simulink model "Final_Model"  (R2022b)
settings: Solver=FixedStepAuto  StartTime=0.0  StopTime=5  FixedStep=0.001  RelTol=1e-3
model workspace: external: MATLAB File F:\Iman\Robotics\Project1\solid_simmmmm\Final_Model_DataFile.m (data not in the file)
undefined symbols (not defined in the file or in its folder): Revolute, Revolute3, Revolute4, smiData, X, Y, Z
libraries: sm_lib x139, nesl_utility x53
(part 4 of 4)

== system Final_Model/IK/Link1_2_RIGID ==
  ReferenceFrame : sm_lib/Frames and Transforms/Reference Frame
  Solid : sm_lib/Body Elements/File Solid  ExtGeomFileName=Link1_Default_sldprt.STEP  UnitType=FromFile  ExtGeomFileUnits=m  StepReaderType=HEX  ExportConvexHullGeometry=off  InertiaType=Custom  Mass=smiData.Solid(3).mass  MassUnits=kg  CenterOfMass=smiData.Solid(3).CoM  CenterOfMassUnits=m  MomentsOfInertia=smiData.Solid(3).MoI  MomentsOfInertiaUnits=kg*m^2  ProductsOfInertia=smiData.Solid(3).PoI  ProductsOfInertiaUnits=kg*m^2  BasedOnType=DensityFromFile  Density=1000  DensityUnits=kg/m^3  DoExposeReferenceFrame=on  SerializedFrames=<Frames/>  GraphicType=FromGeometry  MarkerShape=Sphere  MarkerSize=10  GraphicVisPropType=SimpleVisualProperties  GraphicDiffuseColor=smiData.Solid(3).color  GraphicSpecularColor=[0.5 0.5 0.5 1.0]  GraphicAmbientColor=[0.15 0.15 0.15 1.0]  GraphicEmissiveColor=[0.0 0.0 0.0 1.0]  GraphicShininess=75  GraphicOpacity=smiData.Solid(3).opacity
  Transform : sm_lib/Frames and Transforms/Rigid Transform  TranslationMethod=Cartesian  TranslationStandardOffset=0  TranslationLengthUnit=cm  TranslationStandardAxis=+Z  TranslationCartesianOffset=smiData.RigidTransform(6).translation  TranslationROffset=0  TranslationROffsetUnits=m  TranslationZOffset=0  TranslationZOffsetUnits=m  TranslationThetaOffset=0  TranslationThetaOffsetUnits=deg  RotationMethod=ArbitraryAxis  RotationAngleUnits=rad  RotationStandardAxis=+Z  RotationAngle=smiData.RigidTransform(6).angle  RotationArbitraryAxis=smiData.RigidTransform(6).axis  FollAlignAxisA=+X  BaseAlignAxisA=+Y  FollAlignAxisB=+Y  BaseAlignAxisB=+Z  RotationSequenceAxes=FollowerAxes  RotationSequence=XYX  RotationSequenceAngles=[0 0 0]  RotationSequenceAnglesUnits=deg  RotationMatrix=[1 0 0; 0 1 0; 0 0 1]  Quaternion=[1 0 0 0]
  Transform1 : sm_lib/Frames and Transforms/Rigid Transform  TranslationMethod=Cartesian  TranslationStandardOffset=0  TranslationLengthUnit=cm  TranslationStandardAxis=+Z  TranslationCartesianOffset=smiData.RigidTransform(7).translation  TranslationROffset=0  TranslationROffsetUnits=m  TranslationZOffset=0  TranslationZOffsetUnits=m  TranslationThetaOffset=0  TranslationThetaOffsetUnits=deg  RotationMethod=ArbitraryAxis  RotationAngleUnits=rad  RotationStandardAxis=+Z  RotationAngle=smiData.RigidTransform(7).angle  RotationArbitraryAxis=smiData.RigidTransform(7).axis  FollAlignAxisA=+X  BaseAlignAxisA=+Y  FollAlignAxisB=+Y  BaseAlignAxisB=+Z  RotationSequenceAxes=FollowerAxes  RotationSequence=XYX  RotationSequenceAngles=[0 0 0]  RotationSequenceAnglesUnits=deg  RotationMatrix=[1 0 0; 0 1 0; 0 0 1]  Quaternion=[1 0 0 0]
  F : PMIOPort  Side=Left
  F1 : PMIOPort  Port=2  Side=Right
  connections:
  Solid/RConn1 -- ReferenceFrame/RConn1 -- Transform/LConn1 -- Transform1/LConn1
  Transform/RConn1 -- F/RConn1
  Transform1/RConn1 -- F1/RConn1

== system Final_Model/IK/Link2_1_RIGID ==
  ReferenceFrame : sm_lib/Frames and Transforms/Reference Frame
  Solid : sm_lib/Body Elements/File Solid  ExtGeomFileName=Link2_Default_sldprt.STEP  UnitType=FromFile  ExtGeomFileUnits=m  StepReaderType=HEX  ExportConvexHullGeometry=off  InertiaType=Custom  Mass=smiData.Solid(4).mass  MassUnits=kg  CenterOfMass=smiData.Solid(4).CoM  CenterOfMassUnits=m  MomentsOfInertia=smiData.Solid(4).MoI  MomentsOfInertiaUnits=kg*m^2  ProductsOfInertia=smiData.Solid(4).PoI  ProductsOfInertiaUnits=kg*m^2  BasedOnType=DensityFromFile  Density=1000  DensityUnits=kg/m^3  DoExposeReferenceFrame=on  SerializedFrames=<Frames/>  GraphicType=FromGeometry  MarkerShape=Sphere  MarkerSize=10  GraphicVisPropType=SimpleVisualProperties  GraphicDiffuseColor=smiData.Solid(4).color  GraphicSpecularColor=[0.5 0.5 0.5 1.0]  GraphicAmbientColor=[0.15 0.15 0.15 1.0]  GraphicEmissiveColor=[0.0 0.0 0.0 1.0]  GraphicShininess=75  GraphicOpacity=smiData.Solid(4).opacity
  Transform : sm_lib/Frames and Transforms/Rigid Transform  TranslationMethod=Cartesian  TranslationStandardOffset=0  TranslationLengthUnit=cm  TranslationStandardAxis=+Z  TranslationCartesianOffset=smiData.RigidTransform(5).translation  TranslationROffset=0  TranslationROffsetUnits=m  TranslationZOffset=0  TranslationZOffsetUnits=m  TranslationThetaOffset=0  TranslationThetaOffsetUnits=deg  RotationMethod=ArbitraryAxis  RotationAngleUnits=rad  RotationStandardAxis=+Z  RotationAngle=smiData.RigidTransform(5).angle  RotationArbitraryAxis=smiData.RigidTransform(5).axis  FollAlignAxisA=+X  BaseAlignAxisA=+Y  FollAlignAxisB=+Y  BaseAlignAxisB=+Z  RotationSequenceAxes=FollowerAxes  RotationSequence=XYX  RotationSequenceAngles=[0 0 0]  RotationSequenceAnglesUnits=deg  RotationMatrix=[1 0 0; 0 1 0; 0 0 1]  Quaternion=[1 0 0 0]
  Transform1 : sm_lib/Frames and Transforms/Rigid Transform  TranslationMethod=Cartesian  TranslationStandardOffset=0  TranslationLengthUnit=cm  TranslationStandardAxis=+Z  TranslationCartesianOffset=smiData.RigidTransform(9).translation  TranslationROffset=0  TranslationROffsetUnits=m  TranslationZOffset=0  TranslationZOffsetUnits=m  TranslationThetaOffset=0  TranslationThetaOffsetUnits=deg  RotationMethod=ArbitraryAxis  RotationAngleUnits=rad  RotationStandardAxis=+Z  RotationAngle=smiData.RigidTransform(9).angle  RotationArbitraryAxis=smiData.RigidTransform(9).axis  FollAlignAxisA=+X  BaseAlignAxisA=+Y  FollAlignAxisB=+Y  BaseAlignAxisB=+Z  RotationSequenceAxes=FollowerAxes  RotationSequence=XYX  RotationSequenceAngles=[0 0 0]  RotationSequenceAnglesUnits=deg  RotationMatrix=[1 0 0; 0 1 0; 0 0 1]  Quaternion=[1 0 0 0]
  F : PMIOPort  Side=Right
  F1 : PMIOPort  Port=2  Side=Right
  connections:
  Solid/RConn1 -- ReferenceFrame/RConn1 -- Transform/LConn1 -- Transform1/LConn1
  Transform/RConn1 -- F/RConn1
  Transform1/RConn1 -- F1/RConn1

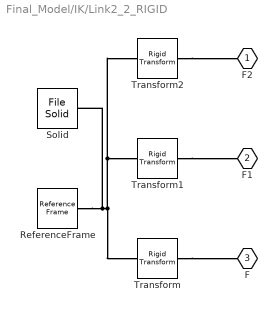
== system Final_Model/IK/Link2_2_RIGID ==
  ReferenceFrame : sm_lib/Frames and Transforms/Reference Frame
  Solid : sm_lib/Body Elements/File Solid  ExtGeomFileName=Link2_Default_sldprt.STEP  UnitType=FromFile  ExtGeomFileUnits=m  StepReaderType=HEX  ExportConvexHullGeometry=off  InertiaType=Custom  Mass=smiData.Solid(4).mass  MassUnits=kg  CenterOfMass=smiData.Solid(4).CoM  CenterOfMassUnits=m  MomentsOfInertia=smiData.Solid(4).MoI  MomentsOfInertiaUnits=kg*m^2  ProductsOfInertia=smiData.Solid(4).PoI  ProductsOfInertiaUnits=kg*m^2  BasedOnType=DensityFromFile  Density=1000  DensityUnits=kg/m^3  DoExposeReferenceFrame=on  SerializedFrames=<Frames/>  GraphicType=FromGeometry  MarkerShape=Sphere  MarkerSize=10  GraphicVisPropType=SimpleVisualProperties  GraphicDiffuseColor=smiData.Solid(4).color  GraphicSpecularColor=[0.5 0.5 0.5 1.0]  GraphicAmbientColor=[0.15 0.15 0.15 1.0]  GraphicEmissiveColor=[0.0 0.0 0.0 1.0]  GraphicShininess=75  GraphicOpacity=smiData.Solid(4).opacity
  Transform : sm_lib/Frames and Transforms/Rigid Transform  TranslationMethod=Cartesian  TranslationStandardOffset=0  TranslationLengthUnit=cm  TranslationStandardAxis=+Z  TranslationCartesianOffset=smiData.RigidTransform(2).translation  TranslationROffset=0  TranslationROffsetUnits=m  TranslationZOffset=0  TranslationZOffsetUnits=m  TranslationThetaOffset=0  TranslationThetaOffsetUnits=deg  RotationMethod=ArbitraryAxis  RotationAngleUnits=rad  RotationStandardAxis=+Z  RotationAngle=smiData.RigidTransform(2).angle  RotationArbitraryAxis=smiData.RigidTransform(2).axis  FollAlignAxisA=+X  BaseAlignAxisA=+Y  FollAlignAxisB=+Y  BaseAlignAxisB=+Z  RotationSequenceAxes=FollowerAxes  RotationSequence=XYX  RotationSequenceAngles=[0 0 0]  RotationSequenceAnglesUnits=deg  RotationMatrix=[1 0 0; 0 1 0; 0 0 1]  Quaternion=[1 0 0 0]
  Transform1 : sm_lib/Frames and Transforms/Rigid Transform  TranslationMethod=Cartesian  TranslationStandardOffset=0  TranslationLengthUnit=cm  TranslationStandardAxis=+Z  TranslationCartesianOffset=smiData.RigidTransform(8).translation  TranslationROffset=0  TranslationROffsetUnits=m  TranslationZOffset=0  TranslationZOffsetUnits=m  TranslationThetaOffset=0  TranslationThetaOffsetUnits=deg  RotationMethod=ArbitraryAxis  RotationAngleUnits=rad  RotationStandardAxis=+Z  RotationAngle=smiData.RigidTransform(8).angle  RotationArbitraryAxis=smiData.RigidTransform(8).axis  FollAlignAxisA=+X  BaseAlignAxisA=+Y  FollAlignAxisB=+Y  BaseAlignAxisB=+Z  RotationSequenceAxes=FollowerAxes  RotationSequence=XYX  RotationSequenceAngles=[0 0 0]  RotationSequenceAnglesUnits=deg  RotationMatrix=[1 0 0; 0 1 0; 0 0 1]  Quaternion=[1 0 0 0]
  Transform2 : sm_lib/Frames and Transforms/Rigid Transform  TranslationMethod=Cartesian  TranslationStandardOffset=0  TranslationLengthUnit=cm  TranslationStandardAxis=+Z  TranslationCartesianOffset=smiData.RigidTransform(11).translation  TranslationROffset=0  TranslationROffsetUnits=m  TranslationZOffset=0  TranslationZOffsetUnits=m  TranslationThetaOffset=0  TranslationThetaOffsetUnits=deg  RotationMethod=ArbitraryAxis  RotationAngleUnits=rad  RotationStandardAxis=+Z  RotationAngle=smiData.RigidTransform(11).angle  RotationArbitraryAxis=smiData.RigidTransform(11).axis  FollAlignAxisA=+X  BaseAlignAxisA=+Y  FollAlignAxisB=+Y  BaseAlignAxisB=+Z  RotationSequenceAxes=FollowerAxes  RotationSequence=XYX  RotationSequenceAngles=[0 0 0]  RotationSequenceAnglesUnits=deg  RotationMatrix=[1 0 0; 0 1 0; 0 0 1]  Quaternion=[1 0 0 0]
  F2 : PMIOPort  Side=Left
  F1 : PMIOPort  Port=2  Side=Left
  F : PMIOPort  Port=3  Side=Left
  connections:
  Solid/RConn1 -- ReferenceFrame/RConn1 -- Transform1/LConn1 -- Transform2/LConn1 -- Transform/LConn1
  Transform/RConn1 -- F/RConn1
  Transform1/RConn1 -- F1/RConn1
  Transform2/RConn1 -- F2/RConn1

== matlab function Final_Model/Rev3 Trajectory/Rev3 trajectories2 ==
  data: t input; theta0 input; pos3 output; thetaf input; thetad0 input; thetadf input; thetadd0 input; thetaddf input; tstart input; pos5 output; tfinal input
function [pos3, pos5] = fcn(t, theta0, thetaf, thetad0, thetadf, thetadd0, thetaddf, tstart, tfinal)
    % Input parameters:
    % t         - current time from Simulink clock
    % theta0    - initial position
    % thetaf    - final position
    % thetad0   - initial velocity
    % thetadf   - final velocity
    % thetadd0  - initial acceleration (for 5th order only)
    % thetaddf  - final acceleration (for 5th order only)
    % tstart    - start time
    % tfinal    - final time
    
    % Outputs:
    % pos3      - position from 3rd order trajectory
    % pos5      - position from 5th order trajectory
    
    % Calculate time duration
    T = tfinal - tstart;
    
    % 3rd order trajectory coefficients
    a0_3 = theta0;
    a1_3 = thetad0;
    a2_3 = (-3 * (theta0 - thetaf) - (2 * thetad0 + thetadf) * T) / T^2;
    a3_3 = (2 * (theta0 - thetaf) + (thetad0 + thetadf) * T) / T^3;
    
    % 5th order trajectory coefficients
    a0_5 = theta0;
    a1_5 = thetad0;
    a2_5 = 0.5 * thetadd0;
    a3_5 = (1/(2*T^3)) * (20 * (thetaf - theta0) - (8 * thetadf + 12*thetad0) * T - (3 * thetaddf - thetadd0) * T^2);
    a4_5 = (1/(2*T^4)) * (30 * (theta0 - thetaf) + (14 * thetadf + 16*thetad0) * T + (3 * thetaddf - 2*thetadd0) * T^2);
    a5_5 = (1/(2*T^5)) * (12 * (thetaf - theta0) - 6*(thetadf + thetad0) * T - (thetaddf - thetadd0) * T^2);
    
    % Calculate relative time
    t_rel = t - tstart;
    
    % Ensure trajectory stays at final position after tfinal
    if t < tstart
        pos3 = theta0;
        pos5 = theta0;
    elseif t > tfinal
        pos3 = thetaf;
        pos5 = thetaf;
    else
        % Calculate positions using polynomial equations
        pos3 = a0_3 + a1_3*t_rel + a2_3*t_rel^2 + a3_3*t_rel^3;
        pos5 = a0_5 + a1_5*t_rel + a2_5*t_rel^2 + a3_5*t_rel^3 + a4_5*t_rel^4 + a5_5*t_rel^5;
    end
end

== matlab function Final_Model/Multiply ==
  data: u input; y1 output; v input; y2 output; y3 output
function [y1, y2, y3] = power(u,v)

y1 = u(1) * v(1);
y2 = u(2) * v(2);
y3 = u(3) * v(3);

== matlab function Final_Model/MATLAB Function1 ==
  data: t input; y output
function y = fcn(t)

y = 30 * sin(t) + 45; %theta2

== matlab function Final_Model/MATLAB Function ==
  data: t input; y output
function y = fcn(t)

y = 30 * sin(t); %theta1

== matlab function Final_Model/MATLAB Function2 ==
  data: t input; y output
function y = fcn(t)

y = 22.5 * sin(t) + 135 ; %theta3

== matlab function Final_Model/MATLAB Function3 ==
  data: t input; y output
function y = fcn(t)

y = 30 * sin(t); %theta1

== matlab function Final_Model/MATLAB Function4 ==
  data: t input; y output
function y = fcn(t)

y = 30 * sin(t) + 45; %theta2

== matlab function Final_Model/MATLAB Function5 ==
  data: t input; y output
function y = fcn(t)

y = 22.5 * sin(t) + 135 ; %theta3

== matlab function Final_Model/MATLAB Function6 ==
  data: x0 input; traj3 output; xf input; v0 input; vf input; a0 input; af input; T input; traj5 output; coeff3 output; coeff5 output; t input
function [traj3, traj5, coeff3, coeff5] = generateTrajectory(x0, xf, v0, vf, a0, af, T,t)
% GENERATETRAJECTORY Generates 3rd and 5th order trajectories.
% 
% Inputs:
%   x0  - Initial position
%   xf  - Final position
%   v0  - Initial velocity
%   vf  - Final velocity
%   a0  - Initial acceleration
%   af  - Final acceleration
%   T   - Total time for the trajectory
%   N   - Number of points for time discretization
% 
% Outputs:
%   traj3  - 3rd order trajectory positions
%   traj5  - 5th order trajectory positions
%   coeff3 - Coefficients of the 3rd order polynomial
%   coeff5 - Coefficients of the 5th order polynomial
%   t      - Time vector
%N = 1;
    % Time vector
    %t = linspace(0, T, N);

    % 3rd-Order Polynomial Coefficients
    A3 = [1, 0, 0, 0; 
          1, T, T^2, T^3; 
          0, 1, 0, 0; 
          0, 1, 2*T, 3*T^2];
    B3 = [x0; xf; v0; vf];
    coeff3 = A3 \ B3;

    % Evaluate 3rd order trajectory
    traj3 = coeff3(1) + coeff3(2)*t + coeff3(3)*t.^2 + coeff3(4)*t.^3;

    % 5th-Order Polynomial Coefficients
    A5 = [1, 0, 0, 0, 0, 0; 
          1, T, T^2, T^3, T^4, T^5; 
          0, 1, 0, 0, 0, 0; 
          0, 1, 2*T, 3*T^2, 4*T^3, 5*T^4; 
          0, 0, 2, 0, 0, 0; 
          0, 0, 2, 6*T, 12*T^2, 20*T^3];
    B5 = [x0; xf; v0; vf; a0; af];
    coeff5 = A5 \ B5;

    % Evaluate 5th order trajectory
    traj5 = coeff5(1) + coeff5(2)*t + coeff5(3)*t.^2 + coeff5(4)*t.^3 + ...
            coeff5(5)*t.^4 + coeff5(6)*t.^5;

%     % Plot the results
%     figure;
%     subplot(2, 1, 1);
%     plot(t, traj3, 'r', 'LineWidth', 2);
%     title('3rd Order Trajectory');
%     xlabel('Time (s)');
%     ylabel('Position (m)');
%     grid on;
% 
%     subplot(2, 1, 2);
%     plot(t, traj5, 'b', 'LineWidth', 2);
%     title('5th Order Trajectory');
%     xlabel('Time (s)');
%     ylabel('Position (m)');
%     grid on;
% 
%     % Display coefficients
%     disp('3rd Order Coefficients:');
%     disp(coeff3);
%     disp('5th Order Coefficients:');
%     disp(coeff5);
end

== matlab function Final_Model/Rev4 Trajectory/Rev4 trajectories ==
  data: t input; theta0 input; pos3 output; thetaf input; thetad0 input; thetadf input; thetadd0 input; thetaddf input; tstart input; pos5 output; tfinal input
function [pos3, pos5] = fcn(t, theta0, thetaf, thetad0, thetadf, thetadd0, thetaddf, tstart, tfinal)
    % Input parameters:
    % t         - current time from Simulink clock
    % theta0    - initial position
    % thetaf    - final position
    % thetad0   - initial velocity
    % thetadf   - final velocity
    % thetadd0  - initial acceleration (for 5th order only)
    % thetaddf  - final acceleration (for 5th order only)
    % tstart    - start time
    % tfinal    - final time
    
    % Outputs:
    % pos3      - position from 3rd order trajectory
    % pos5      - position from 5th order trajectory
    
    % Calculate time duration
    T = tfinal - tstart;
    
    % 3rd order trajectory coefficients
    a0_3 = theta0;
    a1_3 = thetad0;
    a2_3 = (-3 * (theta0 - thetaf) - (2 * thetad0 + thetadf) * T) / T^2;
    a3_3 = (2 * (theta0 - thetaf) + (thetad0 + thetadf) * T) / T^3;
    
    % 5th order trajectory coefficients
    a0_5 = theta0;
    a1_5 = thetad0;
    a2_5 = 0.5 * thetadd0;
    a3_5 = (1/(2*T^3)) * (20 * (thetaf - theta0) - (8 * thetadf + 12*thetad0) * T - (3 * thetaddf - thetadd0) * T^2);
    a4_5 = (1/(2*T^4)) * (30 * (theta0 - thetaf) + (14 * thetadf + 16*thetad0) * T + (3 * thetaddf - 2*thetadd0) * T^2);
    a5_5 = (1/(2*T^5)) * (12 * (thetaf - theta0) - 6*(thetadf + thetad0) * T - (thetaddf - thetadd0) * T^2);
    
    % Calculate relative time
    t_rel = t - tstart;
    
    % Ensure trajectory stays at final position after tfinal
    if t < tstart
        pos3 = theta0;
        pos5 = theta0;
    elseif t > tfinal
        pos3 = thetaf;
        pos5 = thetaf;
    else
        % Calculate positions using polynomial equations
        pos3 = a0_3 + a1_3*t_rel + a2_3*t_rel^2 + a3_3*t_rel^3;
        pos5 = a0_5 + a1_5*t_rel + a2_5*t_rel^2 + a3_5*t_rel^3 + a4_5*t_rel^4 + a5_5*t_rel^5;
    end
end

== matlab function Final_Model/Rev Trajectory/Rev trajectories ==
  data: t input; theta0 input; pos3 output; thetaf input; thetad0 input; thetadf input; thetadd0 input; thetaddf input; tstart input; pos5 output; tfinal input
function [pos3, pos5] = fcn(t, theta0, thetaf, thetad0, thetadf, thetadd0, thetaddf, tstart, tfinal)
    % Input parameters:
    % t         - current time from Simulink clock
    % theta0    - initial position
    % thetaf    - final position
    % thetad0   - initial velocity
    % thetadf   - final velocity
    % thetadd0  - initial acceleration (for 5th order only)
    % thetaddf  - final acceleration (for 5th order only)
    % tstart    - start time
    % tfinal    - final time
    
    % Outputs:
    % pos3      - position from 3rd order trajectory
    % pos5      - position from 5th order trajectory
    
    % Calculate time duration
    T = tfinal - tstart;
    
    % 3rd order trajectory coefficients
    a0_3 = theta0;
    a1_3 = thetad0;
    a2_3 = (-3 * (theta0 - thetaf) - (2 * thetad0 + thetadf) * T) / T^2;
    a3_3 = (2 * (theta0 - thetaf) + (thetad0 + thetadf) * T) / T^3;
    
    % 5th order trajectory coefficients
    a0_5 = theta0;
    a1_5 = thetad0;
    a2_5 = 0.5 * thetadd0;
    a3_5 = (1/(2*T^3)) * (20 * (thetaf - theta0) - (8 * thetadf + 12*thetad0) * T - (3 * thetaddf - thetadd0) * T^2);
    a4_5 = (1/(2*T^4)) * (30 * (theta0 - thetaf) + (14 * thetadf + 16*thetad0) * T + (3 * thetaddf - 2*thetadd0) * T^2);
    a5_5 = (1/(2*T^5)) * (12 * (thetaf - theta0) - 6*(thetadf + thetad0) * T - (thetaddf - thetadd0) * T^2);
    
    % Calculate relative time
    t_rel = t - tstart;
    
    % Ensure trajectory stays at final position after tfinal
    if t < tstart
        pos3 = theta0;
        pos5 = theta0;
    elseif t > tfinal
        pos3 = thetaf;
        pos5 = thetaf;
    else
        % Calculate positions using polynomial equations
        pos3 = a0_3 + a1_3*t_rel + a2_3*t_rel^2 + a3_3*t_rel^3;
        pos5 = a0_5 + a1_5*t_rel + a2_5*t_rel^2 + a3_5*t_rel^3 + a4_5*t_rel^4 + a5_5*t_rel^5;
    end
end
